simulink subsystem "quatFix"  (R2024b)
settings: Solver=VariableStepAuto  StartTime=0.0  StopTime=10.0  RelTol=1e-3
libraries: simulink x1
settings Model: Creator=ricca  LastModifiedBy=ricca

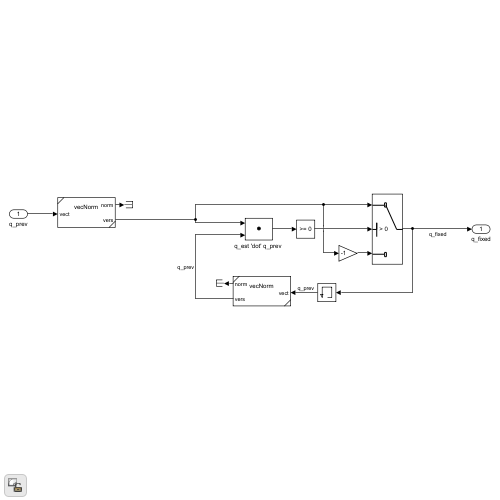
[thumbnail: Simulink's stored preview of the top-level diagram]
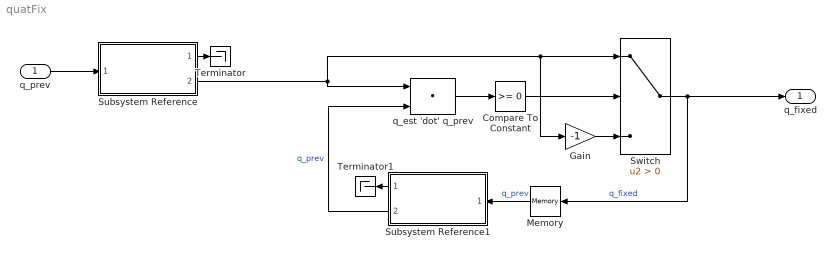
== system quatFix ==
  q_prev : Inport
  Compare To Constant : simulink/Logic and Bit Operations/Compare To Constant  relop=>=  const=0  OutDataTypeStr=boolean
  Gain : Gain  Gain=-1
  Memory : Memory
  Subsystem Reference : Subsystem  ReferencedSubsystem=vecNorm
  Subsystem Reference1 : Subsystem  ReferencedSubsystem=vecNorm
  Switch : Switch  Criteria=u2 > Threshold  SaturateOnIntegerOverflow=off  InputSameDT=off
  Terminator : Terminator
  Terminator1 : Terminator
  "q_est 'dot' q_prev " : DotProduct  OutDataTypeStr=Inherit: Inherit via internal rule
  q_fixed : Outport
  wires:
  q_prev/1 -> Subsystem Reference/1
  Subsystem Reference/1 -> Terminator/1
  Subsystem Reference/2 -> Gain/1, Switch/1, "q_est 'dot' q_prev "/1
  Subsystem Reference1/2 -> "q_est 'dot' q_prev "/2  "q_prev"
  "q_est 'dot' q_prev "/1 -> Compare To Constant/1
  Compare To Constant/1 -> Switch/2
  Switch/1 -> q_fixed/1, Memory/1  "q_fixed"
  Gain/1 -> Switch/3
  Memory/1 -> Subsystem Reference1/1  "q_prev"
  Subsystem Reference1/1 -> Terminator1/1
